simulink model "model"  (R2023b)
settings: Solver=VariableStepAuto  StartTime=0.0  StopTime=10.0  RelTol=1e-3
undefined symbols (not defined in the file): DiscIntNeverNeededParam, Newton, Raphson
libraries: simulink x77, slpidlib x18
(part 3 of 3)

== system model/cfblk32/cfblk14 ==
  cfblk1 : Inport
  cfblk9 : Inport  Port=2
  cfblk10 : Inport  Port=3
  cfblk11 : Inport  Port=4
  cfblk15 : Delay  SampleTime=1
  cfblk3 : simulink/Discrete/Transfer Fcn Lead or Lag  PoleZ=0.95  ZeroZ=0.75  ICPrevOutput=0.0  ICPrevInput=0.0  DoSatur=off
  cfblk4 : slpidlib/PID Controller (2DOF)  Controller=PID  Form=Parallel  TimeDomain=Discrete-time  UseExternalTs=off  SampleTime=1  IntegratorMethod=Forward Euler  FilterMethod=Forward Euler  ControllerParametersSource=internal  P=1  I=1  UseKiTs=off  D=0  N=100  UseFilter=on  b=1  c=1  TunerSelectOption=Transfer Function Based (PID Tuner App)  InitialConditionSource=internal  InitialConditionForIntegrator=0  InitialConditionForFilter=0  DifferentiatorICPrevScaledInput=0  ExternalReset=none  TrackingMode=off  Kt=1  LimitOutput=off  SatLimitsSource=internal  UpperSaturationLimit=inf  LowerSaturationLimit=-inf  LinearizeAsGain=off  AntiWindupMode=none  Kb=1  LimitIntegrator=off  UpperIntegratorSaturationLimit=inf  LowerIntegratorSaturationLimit=-inf  POutMin=[]  POutMax=[]  IOutMin=[]  IOutMax=[]  DOutMin=[]  DOutMax=[]  NOutMin=[]  NOutMax=[]  bOutMin=[]  bOutMax=[]  cOutMin=[]  cOutMax=[]  SumOutMin=[]  SumOutMax=[]  SaturationOutMin=[]  SaturationOutMax=[]  PParamMin=[]  PParamMax=[]  IParamMin=[]  IParamMax=[]  DParamMin=[]  DParamMax=[]  NParamMin=[]  NParamMax=[]  bParamMin=[]  bParamMax=[]  cParamMin=[]  cParamMax=[]  KbParamMin=[]  KbParamMax=[]  KtParamMin=[]  KtParamMax=[]  KbOutMin=[]  KbOutMax=[]  KtOutMin=[]  KtOutMax=[]  IntegratorOutMin=[]  IntegratorOutMax=[]  FilterOutMin=[]  FilterOutMax=[]  SumI1OutMin=[]  SumI1OutMax=[]  SumI2OutMin=[]  SumI2OutMax=[]  SumI3OutMin=[]  SumI3OutMax=[]  SumI4OutMin=[]  SumI4OutMax=[]  SumDOutMin=[]  SumDOutMax=[]  Sum1OutMin=[]  Sum1OutMax=[]  Sum2OutMin=[]  Sum2OutMax=[]  Sum3OutMin=[]  Sum3OutMax=[]  DifferentiatorOutMin=[]  DifferentiatorOutMax=[]  FilterDiffOutCoefMin=[]  FilterDiffOutCoefMax=[]  ReciprocalOutMin=[]  ReciprocalOutMax=[]  SumDenOutMin=[]  SumDenOutMax=[]  SumNumOutMin=[]  SumNumOutMax=[]  DivideOutMin=[]  DivideOutMax=[]  UdiffTsProdOutMin=[]  UdiffTsProdOutMax=[]  NTsProdOutMin=[]  NTsProdOutMax=[]  UintegralTsProdOutMin=[]  UintegralTsProdOutMax=[]  UngainTsProdOutMin=[]  UngainTsProdOutMax=[]  ClampingZeroOutDataTypeStr=Inherit: Inherit via back propagation  ClampingZeroOutMin=[]  ClampingZeroOutMax=[]  FilterDenConstantOutDataTypeStr=Inherit: Inherit via back propagation  FilterDenConstantOutMin=[]  FilterDenConstantOutMax=[]  PCopyOutDataTypeStr=Inherit: Inherit via back propagation  PCopyOutMin=[]  PCopyOutMax=[]  NCopyOutDataTypeStr=Inherit: Inherit via back propagation  NCopyOutMin=[]  NCopyOutMax=[]  IntegratorContinuousStateAttributes=''  IntegratorStateMustResolveToSignalObject=off  IntegratorRTWStateStorageClass=Auto  FilterContinuousStateAttributes=''  FilterStateMustResolveToSignalObject=off  FilterRTWStateStorageClass=Auto  ParallelPVariant=InternalParameters  IdealPVariant=Disabled  IVariant=InternalParameters  DVariant=InternalParameters  bVariant=InternalParameters  cVariant=InternalParameters  IntegratorVariant=Discrete  SatVariant=Disabled  AWVariant=Passthrough  PCopyVariant=Disabled  TRVariant=Disabled  FdbkBlocksVariant=Forward  IdealPFdbkVariant=Disabled  SatFdbkVariant=Disabled  DerivativeFilterVariant=ForwardEulerFilter  NVariant=InternalParameters  NCopyVariant=Disabled  FilterICVariant=InternalICsFilter  IntegratorICVariant=InternalICs  ExternalResetVariant=Disabled  TRSumVariant=Passthrough  SumFdbkVariant=Disabled  SumVariant=Sum_PID  TsampFilterVariant=InternalTs  TsampNgainVariant=Passthrough  TsampIntegralVariant=Disabled_SignalSpec  ExternalSaturationOutDataTypeStr=Inherit: Same as second input
      settings: LibrarySourceBlock=simulink/Discrete/Discrete PID Controller (2DOF)
  cfblk5 : Sin  TimeSource=Use external signal  SampleTime=0
  cfblk6 : Math  Operator=transpose
  cfblk7 : Product
  cfblk8 : Constant  Value=[-199593818.818905]  SampleTime=1
  cfblk2 : Outport
  cfblk12 : Outport  Port=2
  cfblk13 : Outport  Port=3
  cfblk14 : Outport  Port=4
  wires:
  cfblk8/1 -> cfblk2/1
  cfblk6/1 -> cfblk5/1, cfblk7/2
  cfblk5/1 -> cfblk14/1
  cfblk1/1 -> cfblk13/1
  cfblk11/1 -> cfblk12/1
  cfblk9/1 -> cfblk4/1
  cfblk4/1 -> cfblk7/1
  cfblk3/1 -> cfblk6/1
  cfblk10/1 -> cfblk4/2
  cfblk7/1 -> cfblk15/1
  cfblk15/1 -> cfblk3/1

== system model/cfblk32/cfblk8 ==
  cfblk1 : Inport
  cfblk10 : Inport  Port=2
  cfblk11 : Inport  Port=3
  cfblk12 : Inport  Port=4
  cfblk13 : Inport  Port=5
  cfblk14 : Inport  Port=6
  cfblk15 : Delay  SampleTime=1
  cfblk3 : PropagationDelay  SampleTime=1
  cfblk4 : simulink/Discrete/Transfer Fcn Lead or Lag  PoleZ=0.95  ZeroZ=0.75  ICPrevOutput=0.0  ICPrevInput=0.0  DoSatur=off
  cfblk5 : simulink/Discrete/Transfer Fcn First Order  PoleZ=0.95  ICPrevOutput=0.0  DoSatur=off
  cfblk6 : simulink/Discrete/Transfer Fcn Lead or Lag  PoleZ=0.95  ZeroZ=0.75  ICPrevOutput=0.0  ICPrevInput=0.0  DoSatur=off
  cfblk7 : Sum  Inputs=|++
  cfblk8 : Rounding
  cfblk9 : ComplexToRealImag
  cfblk2 : Outport
  wires:
  cfblk12/1 -> cfblk2/1
  cfblk4/1 -> cfblk6/1
  cfblk14/1 -> cfblk8/1
  cfblk11/1 -> cfblk5/1
  cfblk7/1 -> cfblk9/1
  cfblk10/1 -> cfblk4/1
  cfblk5/1 -> cfblk7/1
  cfblk8/1 -> cfblk3/1
  cfblk9/2 -> cfblk3/2
  cfblk9/1 -> cfblk15/1
  cfblk15/1 -> cfblk7/2

== system model/cfblk32/cfblk9 ==
  cfblk1 : Inport
  cfblk5 : Inport  Port=2
  cfblk6 : Inport  Port=3
  cfblk3 : DotProduct  OutDataTypeStr=Inherit: Inherit via internal rule
  cfblk4 : Product  Inputs=**
  cfblk8 : Delay  SampleTime=1
  cfblk2 : Outport
  cfblk7 : Outport  Port=2
  wires:
  cfblk5/1 -> cfblk4/1
  cfblk3/1 -> cfblk4/2, cfblk7/1
  cfblk1/1 -> cfblk2/1
  cfblk6/1 -> cfblk3/1
  cfblk4/1 -> cfblk8/1
  cfblk8/1 -> cfblk3/2

== system model/cfblk35/cfblk10 ==
  cfblk1 : Inport
  cfblk10 : Inport  Port=2
  cfblk11 : Inport  Port=3
  cfblk12 : Inport  Port=4
  cfblk13 : Inport  Port=5
  cfblk3 : DiscreteZeroPole  Poles=[0 0.5]  Gain=1  SampleTime=-1
  cfblk4 : DiscreteStateSpace  SampleTime=-1
  cfblk5 : simulink/Math Operations/Slider Gain  gain=1  low=0  high=2
  cfblk6 : Sin  TimeSource=Use external signal  SampleTime=0
  cfblk7 : Constant  Value=[-112437375.894826]  SampleTime=1
  cfblk8 : Constant  Value=[-453137305.741607]  SampleTime=1
  cfblk9 : Constant  Value=[-741340996.395799]  SampleTime=1
  cfblk2 : Outport
  wires:
  cfblk13/1 -> cfblk6/1
  cfblk5/1 -> cfblk2/1
  cfblk12/1 -> cfblk4/1
  cfblk4/1 -> cfblk3/1
  cfblk6/1 -> cfblk5/1

== system model/cfblk35/cfblk11 ==
  cfblk1 : Inport
  cfblk12 : Inport  Port=2
  cfblk10 : UnaryMinus
  cfblk11 : Squeeze
  cfblk14 : Delay
  cfblk3 : simulink/Discrete/Transfer Fcn Real Zero  ZeroZ=0.75  ICPrevInput=0.0  DoSatur=off
  cfblk4 : DiscreteFir
  cfblk5 : Delay  DelayLengthSource=Input port
      settings: InputPortMap=u0,p1
  cfblk6 : DiscreteStateSpace  SampleTime=-1
  cfblk7 : simulink/Discrete/Transfer Fcn First Order  PoleZ=0.95  ICPrevOutput=0.0  DoSatur=off
  cfblk8 : Reshape
  cfblk9 : simulink/Math Operations/Slider Gain  gain=1  low=0  high=2
  cfblk2 : Outport
  cfblk13 : Outport  Port=2
  wires:
  cfblk4/1 -> cfblk8/1
  cfblk8/1 -> cfblk2/1
  cfblk1/1 -> cfblk10/1
  cfblk3/1 -> cfblk5/1
  cfblk10/1 -> cfblk4/1
  cfblk7/1 -> cfblk9/1
  cfblk11/1 -> cfblk13/1, cfblk6/1
  cfblk12/1 -> cfblk7/1
  cfblk9/1 -> cfblk11/1
  cfblk6/1 -> cfblk5/2
  cfblk5/1 -> cfblk14/1
  cfblk14/1 -> cfblk3/1

== system model/cfblk35/cfblk14 ==
  cfblk1 : Inport
  cfblk5 : Inport  Port=2
  cfblk6 : Inport  Port=3
  Action Port : ActionPort  ActionPortLabel=if(u1 >= 0)
  cfblk3 : DiscreteZeroPole  Poles=[0 0.5]  Gain=1  SampleTime=-1
  cfblk4 : Signum
  cfblk2 : Outport
  cfblk7 : Outport  Port=2
  wires:
  cfblk4/1 -> cfblk3/1
  cfblk5/1 -> cfblk7/1
  cfblk1/1 -> cfblk2/1
  cfblk6/1 -> cfblk4/1

== system model/cfblk35/cfblk15 ==
  cfblk1 : Inport
  Action Port : ActionPort  ActionPortLabel=else
  cfblk10 : Signum
  cfblk11 : Math
  cfblk12 : Bias  Bias=[228101489.768927]  SaturateOnIntegerOverflow=off
  cfblk13 : Constant  Value=[208020800.146715]  SampleTime=1
  cfblk16 : Delay
  cfblk3 : DiscreteStateSpace  SampleTime=-1
  cfblk4 : slpidlib/PID Controller (2DOF)  Controller=PID  Form=Parallel  TimeDomain=Discrete-time  UseExternalTs=off  SampleTime=-1  IntegratorMethod=Forward Euler  FilterMethod=Forward Euler  ControllerParametersSource=internal  P=1  I=1  UseKiTs=off  D=0  N=100  UseFilter=on  b=1  c=1  TunerSelectOption=Transfer Function Based (PID Tuner App)  InitialConditionSource=internal  InitialConditionForIntegrator=0  InitialConditionForFilter=0  DifferentiatorICPrevScaledInput=0  ExternalReset=none  TrackingMode=off  Kt=1  LimitOutput=off  SatLimitsSource=internal  UpperSaturationLimit=inf  LowerSaturationLimit=-inf  LinearizeAsGain=off  AntiWindupMode=none  Kb=1  LimitIntegrator=off  UpperIntegratorSaturationLimit=inf  LowerIntegratorSaturationLimit=-inf  POutMin=[]  POutMax=[]  IOutMin=[]  IOutMax=[]  DOutMin=[]  DOutMax=[]  NOutMin=[]  NOutMax=[]  bOutMin=[]  bOutMax=[]  cOutMin=[]  cOutMax=[]  SumOutMin=[]  SumOutMax=[]  SaturationOutMin=[]  SaturationOutMax=[]  PParamMin=[]  PParamMax=[]  IParamMin=[]  IParamMax=[]  DParamMin=[]  DParamMax=[]  NParamMin=[]  NParamMax=[]  bParamMin=[]  bParamMax=[]  cParamMin=[]  cParamMax=[]  KbParamMin=[]  KbParamMax=[]  KtParamMin=[]  KtParamMax=[]  KbOutMin=[]  KbOutMax=[]  KtOutMin=[]  KtOutMax=[]  IntegratorOutMin=[]  IntegratorOutMax=[]  FilterOutMin=[]  FilterOutMax=[]  SumI1OutMin=[]  SumI1OutMax=[]  SumI2OutMin=[]  SumI2OutMax=[]  SumI3OutMin=[]  SumI3OutMax=[]  SumI4OutMin=[]  SumI4OutMax=[]  SumDOutMin=[]  SumDOutMax=[]  Sum1OutMin=[]  Sum1OutMax=[]  Sum2OutMin=[]  Sum2OutMax=[]  Sum3OutMin=[]  Sum3OutMax=[]  DifferentiatorOutMin=[]  DifferentiatorOutMax=[]  FilterDiffOutCoefMin=[]  FilterDiffOutCoefMax=[]  ReciprocalOutMin=[]  ReciprocalOutMax=[]  SumDenOutMin=[]  SumDenOutMax=[]  SumNumOutMin=[]  SumNumOutMax=[]  DivideOutMin=[]  DivideOutMax=[]  UdiffTsProdOutMin=[]  UdiffTsProdOutMax=[]  NTsProdOutMin=[]  NTsProdOutMax=[]  UintegralTsProdOutMin=[]  UintegralTsProdOutMax=[]  UngainTsProdOutMin=[]  UngainTsProdOutMax=[]  ClampingZeroOutDataTypeStr=Inherit: Inherit via back propagation  ClampingZeroOutMin=[]  ClampingZeroOutMax=[]  FilterDenConstantOutDataTypeStr=Inherit: Inherit via back propagation  FilterDenConstantOutMin=[]  FilterDenConstantOutMax=[]  PCopyOutDataTypeStr=Inherit: Inherit via back propagation  PCopyOutMin=[]  PCopyOutMax=[]  NCopyOutDataTypeStr=Inherit: Inherit via back propagation  NCopyOutMin=[]  NCopyOutMax=[]  IntegratorContinuousStateAttributes=''  IntegratorStateMustResolveToSignalObject=off  IntegratorRTWStateStorageClass=Auto  FilterContinuousStateAttributes=''  FilterStateMustResolveToSignalObject=off  FilterRTWStateStorageClass=Auto  ParallelPVariant=InternalParameters  IdealPVariant=Disabled  IVariant=InternalParameters  DVariant=InternalParameters  bVariant=InternalParameters  cVariant=InternalParameters  IntegratorVariant=Discrete  SatVariant=Disabled  AWVariant=Passthrough  PCopyVariant=Disabled  TRVariant=Disabled  FdbkBlocksVariant=Forward  IdealPFdbkVariant=Disabled  SatFdbkVariant=Disabled  DerivativeFilterVariant=ForwardEulerFilter  NVariant=InternalParameters  NCopyVariant=Disabled  FilterICVariant=InternalICsFilter  IntegratorICVariant=InternalICs  ExternalResetVariant=Disabled  TRSumVariant=Passthrough  SumFdbkVariant=Disabled  SumVariant=Sum_PID  TsampFilterVariant=InternalTs  TsampNgainVariant=Passthrough  TsampIntegralVariant=Disabled_SignalSpec  ExternalSaturationOutDataTypeStr=Inherit: Same as second input
      settings: LibrarySourceBlock=simulink/Discrete/Discrete PID Controller (2DOF)
  cfblk5 : slpidlib/PID Controller  Controller=PID  Form=Parallel  TimeDomain=Discrete-time  UseExternalTs=off  SampleTime=-1  IntegratorMethod=Forward Euler  FilterMethod=Forward Euler  ControllerParametersSource=internal  P=1  I=1  UseKiTs=off  D=0  N=100  UseFilter=on  TunerSelectOption=Transfer Function Based (PID Tuner App)  InitialConditionSource=internal  InitialConditionForIntegrator=0  InitialConditionForFilter=0  DifferentiatorICPrevScaledInput=0  ExternalReset=none  TrackingMode=off  Kt=1  LimitOutput=off  SatLimitsSource=internal  UpperSaturationLimit=inf  LowerSaturationLimit=-inf  LinearizeAsGain=off  AntiWindupMode=none  Kb=1  LimitIntegrator=off  UpperIntegratorSaturationLimit=inf  LowerIntegratorSaturationLimit=-inf  POutMin=[]  POutMax=[]  IOutMin=[]  IOutMax=[]  DOutMin=[]  DOutMax=[]  NOutMin=[]  NOutMax=[]  SumOutMin=[]  SumOutMax=[]  SaturationOutMin=[]  SaturationOutMax=[]  PParamMin=[]  PParamMax=[]  IParamMin=[]  IParamMax=[]  DParamMin=[]  DParamMax=[]  NParamMin=[]  NParamMax=[]  KbParamMin=[]  KbParamMax=[]  KtParamMin=[]  KtParamMax=[]  KbOutMin=[]  KbOutMax=[]  KtOutMin=[]  KtOutMax=[]  IntegratorOutMin=[]  IntegratorOutMax=[]  FilterOutMin=[]  FilterOutMax=[]  SumI1OutMin=[]  SumI1OutMax=[]  SumI2OutMin=[]  SumI2OutMax=[]  SumI3OutMin=[]  SumI3OutMax=[]  SumI4OutMin=[]  SumI4OutMax=[]  SumDOutMin=[]  SumDOutMax=[]  DifferentiatorOutMin=[]  DifferentiatorOutMax=[]  FilterDiffOutCoefMin=[]  FilterDiffOutCoefMax=[]  ReciprocalOutMin=[]  ReciprocalOutMax=[]  SumDenOutMin=[]  SumDenOutMax=[]  SumNumOutMin=[]  SumNumOutMax=[]  DivideOutMin=[]  DivideOutMax=[]  UdiffTsProdOutMin=[]  UdiffTsProdOutMax=[]  NTsProdOutMin=[]  NTsProdOutMax=[]  UintegralTsProdOutMin=[]  UintegralTsProdOutMax=[]  UngainTsProdOutMin=[]  UngainTsProdOutMax=[]  ClampingZeroOutDataTypeStr=Inherit: Inherit via back propagation  ClampingZeroOutMin=[]  ClampingZeroOutMax=[]  FilterDenConstantOutDataTypeStr=Inherit: Inherit via back propagation  FilterDenConstantOutMin=[]  FilterDenConstantOutMax=[]  PCopyOutDataTypeStr=Inherit: Inherit via back propagation  PCopyOutMin=[]  PCopyOutMax=[]  NCopyOutDataTypeStr=Inherit: Inherit via back propagation  NCopyOutMin=[]  NCopyOutMax=[]  IntegratorContinuousStateAttributes=''  IntegratorStateMustResolveToSignalObject=off  IntegratorRTWStateStorageClass=Auto  FilterContinuousStateAttributes=''  FilterStateMustResolveToSignalObject=off  FilterRTWStateStorageClass=Auto  ParallelPVariant=InternalParameters  IdealPVariant=Disabled  IVariant=InternalParameters  DVariant=InternalParameters  IntegratorVariant=Discrete  SatVariant=Disabled  AWVariant=Passthrough  PCopyVariant=Disabled  TRVariant=Disabled  FdbkBlocksVariant=Forward  IdealPFdbkVariant=Disabled  SatFdbkVariant=Disabled  DerivativeFilterVariant=ForwardEulerFilter  NVariant=InternalParameters  NCopyVariant=Disabled  FilterICVariant=InternalICsFilter  IntegratorICVariant=InternalICs  ExternalResetVariant=Disabled  TRSumVariant=Passthrough  SumFdbkVariant=Disabled  SumVariant=Sum_PID  TsampFilterVariant=InternalTs  TsampNgainVariant=Passthrough  TsampIntegralVariant=Disabled_SignalSpec  ExternalSaturationOutDataTypeStr=Inherit: Same as second input
      settings: LibrarySourceBlock=simulink/Discrete/Discrete PID Controller
  cfblk6 : DiscreteZeroPole  Poles=[0 0.5]  Gain=1  SampleTime=-1
  cfblk7 : UnitDelay  SampleTime=-1  HasFrameUpgradeWarning=on
  cfblk8 : slpidlib/PID Controller  Controller=PID  Form=Parallel  TimeDomain=Discrete-time  UseExternalTs=off  SampleTime=-1  IntegratorMethod=Forward Euler  FilterMethod=Forward Euler  ControllerParametersSource=internal  P=1  I=1  UseKiTs=off  D=0  N=100  UseFilter=on  TunerSelectOption=Transfer Function Based (PID Tuner App)  InitialConditionSource=internal  InitialConditionForIntegrator=0  InitialConditionForFilter=0  DifferentiatorICPrevScaledInput=0  ExternalReset=none  TrackingMode=off  Kt=1  LimitOutput=off  SatLimitsSource=internal  UpperSaturationLimit=inf  LowerSaturationLimit=-inf  LinearizeAsGain=off  AntiWindupMode=none  Kb=1  LimitIntegrator=off  UpperIntegratorSaturationLimit=inf  LowerIntegratorSaturationLimit=-inf  POutMin=[]  POutMax=[]  IOutMin=[]  IOutMax=[]  DOutMin=[]  DOutMax=[]  NOutMin=[]  NOutMax=[]  SumOutMin=[]  SumOutMax=[]  SaturationOutMin=[]  SaturationOutMax=[]  PParamMin=[]  PParamMax=[]  IParamMin=[]  IParamMax=[]  DParamMin=[]  DParamMax=[]  NParamMin=[]  NParamMax=[]  KbParamMin=[]  KbParamMax=[]  KtParamMin=[]  KtParamMax=[]  KbOutMin=[]  KbOutMax=[]  KtOutMin=[]  KtOutMax=[]  IntegratorOutMin=[]  IntegratorOutMax=[]  FilterOutMin=[]  FilterOutMax=[]  SumI1OutMin=[]  SumI1OutMax=[]  SumI2OutMin=[]  SumI2OutMax=[]  SumI3OutMin=[]  SumI3OutMax=[]  SumI4OutMin=[]  SumI4OutMax=[]  SumDOutMin=[]  SumDOutMax=[]  DifferentiatorOutMin=[]  DifferentiatorOutMax=[]  FilterDiffOutCoefMin=[]  FilterDiffOutCoefMax=[]  ReciprocalOutMin=[]  ReciprocalOutMax=[]  SumDenOutMin=[]  SumDenOutMax=[]  SumNumOutMin=[]  SumNumOutMax=[]  DivideOutMin=[]  DivideOutMax=[]  UdiffTsProdOutMin=[]  UdiffTsProdOutMax=[]  NTsProdOutMin=[]  NTsProdOutMax=[]  UintegralTsProdOutMin=[]  UintegralTsProdOutMax=[]  UngainTsProdOutMin=[]  UngainTsProdOutMax=[]  ClampingZeroOutDataTypeStr=Inherit: Inherit via back propagation  ClampingZeroOutMin=[]  ClampingZeroOutMax=[]  FilterDenConstantOutDataTypeStr=Inherit: Inherit via back propagation  FilterDenConstantOutMin=[]  FilterDenConstantOutMax=[]  PCopyOutDataTypeStr=Inherit: Inherit via back propagation  PCopyOutMin=[]  PCopyOutMax=[]  NCopyOutDataTypeStr=Inherit: Inherit via back propagation  NCopyOutMin=[]  NCopyOutMax=[]  IntegratorContinuousStateAttributes=''  IntegratorStateMustResolveToSignalObject=off  IntegratorRTWStateStorageClass=Auto  FilterContinuousStateAttributes=''  FilterStateMustResolveToSignalObject=off  FilterRTWStateStorageClass=Auto  ParallelPVariant=InternalParameters  IdealPVariant=Disabled  IVariant=InternalParameters  DVariant=InternalParameters  IntegratorVariant=Discrete  SatVariant=Disabled  AWVariant=Passthrough  PCopyVariant=Disabled  TRVariant=Disabled  FdbkBlocksVariant=Forward  IdealPFdbkVariant=Disabled  SatFdbkVariant=Disabled  DerivativeFilterVariant=ForwardEulerFilter  NVariant=InternalParameters  NCopyVariant=Disabled  FilterICVariant=InternalICsFilter  IntegratorICVariant=InternalICs  ExternalResetVariant=Disabled  TRSumVariant=Passthrough  SumFdbkVariant=Disabled  SumVariant=Sum_PID  TsampFilterVariant=InternalTs  TsampNgainVariant=Passthrough  TsampIntegralVariant=Disabled_SignalSpec  ExternalSaturationOutDataTypeStr=Inherit: Same as second input
      settings: LibrarySourceBlock=simulink/Discrete/Discrete PID Controller
  cfblk9 : Sqrt  Operator=rSqrt  AlgorithmType=Newton-Raphson
  cfblk2 : Outport
  cfblk14 : Outport  Port=2
  cfblk15 : Outport  Port=3
  wires:
  cfblk6/1 -> cfblk4/1
  cfblk4/1 -> cfblk10/1
  cfblk1/1 -> cfblk5/1, cfblk9/1
  cfblk5/1 -> cfblk15/1, cfblk14/1
  cfblk9/1 -> cfblk2/1
  cfblk13/1 -> cfblk4/2
  cfblk12/1 -> cfblk7/1
  cfblk10/1 -> cfblk11/1
  cfblk8/1 -> cfblk6/1
  cfblk3/1 -> cfblk8/1
  cfblk11/1 -> cfblk12/1
  cfblk7/1 -> cfblk16/1
  cfblk16/1 -> cfblk3/1

== system model/cfblk35/cfblk9 ==
  cfblk1 : Inport
  cfblk8 : Inport  Port=2
  cfblk9 : Inport  Port=3
  cfblk10 : Inport  Port=4
  cfblk3 : PermuteDimensions
  cfblk4 : Sum  Inputs=+-
  cfblk5 : Sin  TimeSource=Use external signal  SampleTime=0
  cfblk6 : Constant  Value=[547262071.975775]  SampleTime=1
  cfblk7 : Constant  Value=[-884998425.678320]  SampleTime=1
  cfblk2 : Outport
  cfblk11 : Outport  Port=2
  wires:
  cfblk5/1 -> cfblk3/1
  cfblk10/1 -> cfblk4/1
  cfblk9/1 -> cfblk5/1
  cfblk1/1 -> cfblk11/1
  cfblk7/1 -> cfblk2/1
  cfblk8/1 -> cfblk4/2

== system model/cfblk36/cfblk6 ==
  cfblk1 : Inport
  cfblk13 : Inport  Port=2
  cfblk10 : simulink/Math Operations/Slider Gain  gain=1  low=0  high=2
  cfblk11 : Polyval  Coefs=[ +2.081618890e-019, -1.441693666e-014, +4.719686976e-010, -8.536869453e-006, +1.621573104e-001, -8.087801117e+001 ]
  cfblk12 : Constant  Value=[-516293650.996945]  SampleTime=1
  cfblk15 : Delay
  cfblk3 : DiscreteZeroPole  Poles=[0 0.5]  Gain=1  SampleTime=-1
  cfblk4 : simulink/Discrete/Transfer Fcn Lead or Lag  PoleZ=0.95  ZeroZ=0.75  ICPrevOutput=0.0  ICPrevInput=0.0  DoSatur=off
  cfblk5 : DiscreteStateSpace  SampleTime=-1
  cfblk6 : ComplexToRealImag
  cfblk7 : Trigonometry
  cfblk8 : Product  Inputs=**
  cfblk9 : PermuteDimensions
  cfblk2 : Outport
  cfblk14 : Outport  Port=2
  wires:
  cfblk11/1 -> cfblk5/1
  cfblk6/1 -> cfblk9/1
  cfblk10/1 -> cfblk7/1
  cfblk12/1 -> cfblk14/1
  cfblk4/1 -> cfblk10/1
  cfblk6/2 -> cfblk3/1
  cfblk1/1 -> cfblk6/1
  cfblk13/1 -> cfblk11/1
  cfblk3/1 -> cfblk2/1
  cfblk9/1 -> cfblk8/1
  cfblk5/1 -> cfblk8/2
  cfblk7/1 -> cfblk15/1
  cfblk15/1 -> cfblk4/1

== system model/cfblk36/cfblk7 ==
  cfblk1 : Inport
  cfblk13 : Inport  Port=2
  cfblk14 : Inport  Port=3
  cfblk10 : ComplexToRealImag
  cfblk11 : Constant  Value=[929504628.332843]  SampleTime=1
  cfblk12 : Constant  Value=[-286290192.988281]  SampleTime=1
  cfblk3 : simulink/Discrete/Transfer Fcn Lead or Lag  PoleZ=0.95  ZeroZ=0.75  ICPrevOutput=0.0  ICPrevInput=0.0  DoSatur=off
  cfblk4 : Reshape
  cfblk5 : Bias  Bias=[-880605367.001001]  SaturateOnIntegerOverflow=off
  cfblk6 : DotProduct  OutDataTypeStr=Inherit: Inherit via internal rule
  cfblk7 : PermuteDimensions
  cfblk8 : simulink/Math Operations/MinMax Running Resettable  Function=min  vinit=0.0
  cfblk9 : Sqrt  Operator=rSqrt  AlgorithmType=Newton-Raphson
  cfblk2 : Outport
  cfblk15 : Outport  Port=2
  wires:
  cfblk1/1 -> cfblk9/1
  cfblk5/1 -> cfblk3/1
  cfblk8/1 -> cfblk2/1
  cfblk14/1 -> cfblk8/1
  cfblk6/1 -> cfblk8/2
  cfblk9/1 -> cfblk6/1
  cfblk11/1 -> cfblk15/1
  cfblk3/1 -> cfblk10/1
  cfblk12/1 -> cfblk7/1
  cfblk7/1 -> cfblk6/2
  cfblk4/1 -> cfblk5/1
  cfblk13/1 -> cfblk4/1

== system model/cfblk36/cfblk8 ==
  cfblk1 : Inport
  cfblk7 : Inport  Port=2
  cfblk8 : Inport  Port=3
  cfblk3 : simulink/Discrete/Transfer Fcn Real Zero  ZeroZ=0.75  ICPrevInput=0.0  DoSatur=off
  cfblk4 : simulink/Discrete/Transfer Fcn Real Zero  ZeroZ=0.75  ICPrevInput=0.0  DoSatur=off
  cfblk5 : Constant  Value=[893736484.888777]  SampleTime=1
  cfblk6 : Constant  Value=[-931401752.986753]  SampleTime=1
  cfblk2 : Outport
  cfblk9 : Outport  Port=2
  wires:
  cfblk3/1 -> cfblk9/1
  cfblk8/1 -> cfblk4/1
  cfblk7/1 -> cfblk2/1
  cfblk6/1 -> cfblk3/1

== system model/cfblk37/cfblk4 ==
  cfblk1 : Inport
  cfblk12 : Inport  Port=2
  cfblk13 : Inport  Port=3
  cfblk14 : Inport  Port=4
  cfblk10 : Constant  Value=[-744076515.280142]  SampleTime=1
  cfblk11 : Constant  Value=[-214790099.930049]  SampleTime=1
  cfblk17 : Delay
  cfblk3 : Delay
  cfblk4 : Reshape
  cfblk5 : UnaryMinus
  cfblk6 : Bias  Bias=[884710916.406855]  SaturateOnIntegerOverflow=off
  cfblk7 : MinMax  Function=max  Inputs=2
  cfblk8 : simulink/Math Operations/Slider Gain  gain=1  low=0  high=2
  cfblk9 : Sqrt  Operator=rSqrt  AlgorithmType=Newton-Raphson
  cfblk2 : Outport
  cfblk15 : Outport  Port=2
  cfblk16 : Outport  Port=3
  wires:
  cfblk12/1 -> cfblk5/1
  cfblk9/1 -> cfblk16/1
  cfblk3/1 -> cfblk15/1
  cfblk6/1 -> cfblk2/1
  cfblk7/1 -> cfblk6/1
  cfblk4/1 -> cfblk8/1
  cfblk10/1 -> cfblk9/1
  cfblk13/1 -> cfblk7/1
  cfblk11/1 -> cfblk7/2
  cfblk5/1 -> cfblk3/1
  cfblk8/1 -> cfblk17/1
  cfblk17/1 -> cfblk4/1

== system model/cfblk37/cfblk5 ==
  cfblk1 : Inport
  cfblk14 : Inport  Port=2
  cfblk10 : Abs  SaturateOnIntegerOverflow=off
  cfblk11 : Sum  Inputs=+
  cfblk12 : Constant  Value=[-34818510.735228]  SampleTime=1
  cfblk13 : Constant  Value=[-645267266.388667]  SampleTime=1
  cfblk3 : Delay  DelayLengthSource=Input port
      settings: InputPortMap=u0,p1
  cfblk4 : simulink/Math Operations/Slider Gain  gain=1  low=0  high=2
  cfblk5 : Squeeze
  cfblk6 : Reshape
  cfblk7 : Signum
  cfblk8 : Sin  TimeSource=Use external signal  SampleTime=0
  cfblk9 : simulink/Math Operations/MinMax Running Resettable  Function=min  vinit=0.0
  cfblk2 : Outport
  cfblk15 : Outport  Port=2
  cfblk16 : Outport  Port=3
  wires:
  cfblk9/1 -> cfblk3/1
  cfblk13/1 -> cfblk10/1
  cfblk3/1 -> cfblk5/1
  cfblk10/1 -> cfblk3/2
  cfblk5/1 -> cfblk2/1
  cfblk11/1 -> cfblk7/1
  cfblk12/1 -> cfblk6/1
  cfblk1/1 -> cfblk11/1
  cfblk14/1 -> cfblk15/1
  cfblk8/1 -> cfblk16/1
  cfblk7/1 -> cfblk8/1
  cfblk6/1 -> cfblk4/1
  cfblk4/1 -> cfblk9/1, cfblk9/2

== system model/cfblk37/cfblk6 ==
  cfblk1 : Inport
  cfblk8 : Inport  Port=2
  cfblk9 : Inport  Port=3
  cfblk10 : Delay
  cfblk3 : Delay  DelayLengthSource=Input port
      settings: InputPortMap=u0,p1
  cfblk4 : simulink/Discrete/Difference  ICPrevInput=0.0  OutMin=[]  OutMax=[]  OutDataTypeStr=Inherit: Inherit via back propagation  OutDataType=fixdt(1, 16)  OutScaling=2^-10  DoSatur=off
  cfblk5 : DiscreteStateSpace  SampleTime=-1
  cfblk6 : Abs  SaturateOnIntegerOverflow=off
  cfblk7 : Constant  Value=[-149473581.259236]  SampleTime=1
  cfblk2 : Outport
  wires:
  cfblk1/1 -> cfblk3/1
  cfblk7/1 -> cfblk4/1
  cfblk9/1 -> cfblk5/1
  cfblk3/1 -> cfblk6/1
  cfblk5/1 -> cfblk2/1
  cfblk6/1 -> cfblk10/1
  cfblk10/1 -> cfblk3/2

== system model/cfblk37/cfblk7 ==
  cfblk1 : Inport
  cfblk5 : Inport  Port=2
  cfblk6 : Inport  Port=3
  cfblk7 : Inport  Port=4
  cfblk3 : simulink/Discrete/Transfer Fcn Lead or Lag  PoleZ=0.95  ZeroZ=0.75  ICPrevOutput=0.0  ICPrevInput=0.0  DoSatur=off
  cfblk4 : Sum
  cfblk2 : Outport
  wires:
  cfblk5/1 -> cfblk4/1
  cfblk6/1 -> cfblk4/2
  cfblk1/1 -> cfblk3/1
  cfblk7/1 -> cfblk2/1

== system model/cfblk38/cfblk10 ==
  cfblk1 : Inport
  cfblk8 : Inport  Port=2
  cfblk3 : Abs  SaturateOnIntegerOverflow=off
  cfblk4 : Sin  TimeSource=Use external signal  SampleTime=0
  cfblk5 : Product  Inputs=**
  cfblk6 : Constant  Value=[-244203584.019798]  SampleTime=1
  cfblk7 : Constant  Value=[-497272579.083426]  SampleTime=1
  cfblk2 : Outport
  cfblk9 : Outport  Port=2
  wires:
  cfblk7/1 -> cfblk3/1
  cfblk6/1 -> cfblk4/1
  cfblk3/1 -> cfblk5/1
  cfblk8/1 -> cfblk2/1
  cfblk4/1 -> cfblk5/2
  cfblk1/1 -> cfblk9/1

== system model/cfblk38/cfblk11 ==
  cfblk1 : Inport
  cfblk9 : Inport  Port=2
  cfblk10 : Inport  Port=3
  cfblk11 : Inport  Port=4
  cfblk12 : Inport  Port=5
  cfblk13 : Inport  Port=6
  cfblk14 : Delay
  cfblk3 : slpidlib/PID Controller  Controller=PID  Form=Parallel  TimeDomain=Discrete-time  UseExternalTs=off  SampleTime=-1  IntegratorMethod=Forward Euler  FilterMethod=Forward Euler  ControllerParametersSource=internal  P=1  I=1  UseKiTs=off  D=0  N=100  UseFilter=on  TunerSelectOption=Transfer Function Based (PID Tuner App)  InitialConditionSource=internal  InitialConditionForIntegrator=0  InitialConditionForFilter=0  DifferentiatorICPrevScaledInput=0  ExternalReset=none  TrackingMode=off  Kt=1  LimitOutput=off  SatLimitsSource=internal  UpperSaturationLimit=inf  LowerSaturationLimit=-inf  LinearizeAsGain=off  AntiWindupMode=none  Kb=1  LimitIntegrator=off  UpperIntegratorSaturationLimit=inf  LowerIntegratorSaturationLimit=-inf  POutMin=[]  POutMax=[]  IOutMin=[]  IOutMax=[]  DOutMin=[]  DOutMax=[]  NOutMin=[]  NOutMax=[]  SumOutMin=[]  SumOutMax=[]  SaturationOutMin=[]  SaturationOutMax=[]  PParamMin=[]  PParamMax=[]  IParamMin=[]  IParamMax=[]  DParamMin=[]  DParamMax=[]  NParamMin=[]  NParamMax=[]  KbParamMin=[]  KbParamMax=[]  KtParamMin=[]  KtParamMax=[]  KbOutMin=[]  KbOutMax=[]  KtOutMin=[]  KtOutMax=[]  IntegratorOutMin=[]  IntegratorOutMax=[]  FilterOutMin=[]  FilterOutMax=[]  SumI1OutMin=[]  SumI1OutMax=[]  SumI2OutMin=[]  SumI2OutMax=[]  SumI3OutMin=[]  SumI3OutMax=[]  SumI4OutMin=[]  SumI4OutMax=[]  SumDOutMin=[]  SumDOutMax=[]  DifferentiatorOutMin=[]  DifferentiatorOutMax=[]  FilterDiffOutCoefMin=[]  FilterDiffOutCoefMax=[]  ReciprocalOutMin=[]  ReciprocalOutMax=[]  SumDenOutMin=[]  SumDenOutMax=[]  SumNumOutMin=[]  SumNumOutMax=[]  DivideOutMin=[]  DivideOutMax=[]  UdiffTsProdOutMin=[]  UdiffTsProdOutMax=[]  NTsProdOutMin=[]  NTsProdOutMax=[]  UintegralTsProdOutMin=[]  UintegralTsProdOutMax=[]  UngainTsProdOutMin=[]  UngainTsProdOutMax=[]  ClampingZeroOutDataTypeStr=Inherit: Inherit via back propagation  ClampingZeroOutMin=[]  ClampingZeroOutMax=[]  FilterDenConstantOutDataTypeStr=Inherit: Inherit via back propagation  FilterDenConstantOutMin=[]  FilterDenConstantOutMax=[]  PCopyOutDataTypeStr=Inherit: Inherit via back propagation  PCopyOutMin=[]  PCopyOutMax=[]  NCopyOutDataTypeStr=Inherit: Inherit via back propagation  NCopyOutMin=[]  NCopyOutMax=[]  IntegratorContinuousStateAttributes=''  IntegratorStateMustResolveToSignalObject=off  IntegratorRTWStateStorageClass=Auto  FilterContinuousStateAttributes=''  FilterStateMustResolveToSignalObject=off  FilterRTWStateStorageClass=Auto  ParallelPVariant=InternalParameters  IdealPVariant=Disabled  IVariant=InternalParameters  DVariant=InternalParameters  IntegratorVariant=Discrete  SatVariant=Disabled  AWVariant=Passthrough  PCopyVariant=Disabled  TRVariant=Disabled  FdbkBlocksVariant=Forward  IdealPFdbkVariant=Disabled  SatFdbkVariant=Disabled  DerivativeFilterVariant=ForwardEulerFilter  NVariant=InternalParameters  NCopyVariant=Disabled  FilterICVariant=InternalICsFilter  IntegratorICVariant=InternalICs  ExternalResetVariant=Disabled  TRSumVariant=Passthrough  SumFdbkVariant=Disabled  SumVariant=Sum_PID  TsampFilterVariant=InternalTs  TsampNgainVariant=Passthrough  TsampIntegralVariant=Disabled_SignalSpec  ExternalSaturationOutDataTypeStr=Inherit: Same as second input
      settings: LibrarySourceBlock=simulink/Discrete/Discrete PID Controller
  cfblk4 : UnitDelay  SampleTime=-1  HasFrameUpgradeWarning=on
  cfblk5 : Rounding
  cfblk6 : Polyval  Coefs=[ +2.081618890e-019, -1.441693666e-014, +4.719686976e-010, -8.536869453e-006, +1.621573104e-001, -8.087801117e+001 ]
  cfblk7 : Sum  Inputs=--
  cfblk8 : Squeeze
  cfblk2 : Outport
  wires:
  cfblk13/1 -> cfblk4/1
  cfblk5/1 -> cfblk8/1
  cfblk6/1 -> cfblk2/1
  cfblk1/1 -> cfblk7/1
  cfblk9/1 -> cfblk7/2
  cfblk4/1 -> cfblk3/1
  cfblk7/1 -> cfblk6/1
  cfblk8/1 -> cfblk14/1
  cfblk14/1 -> cfblk5/1

== system model/cfblk38/cfblk12 ==
  cfblk1 : Inport
  cfblk10 : Inport  Port=2
  cfblk11 : Inport  Port=3
  cfblk15 : Delay
  cfblk3 : Delay  DelayLengthSource=Input port
      settings: InputPortMap=u0,p1
  cfblk4 : Delay  DelayLengthSource=Input port
      settings: InputPortMap=u0,p1
  cfblk5 : simulink/Discrete/Difference  ICPrevInput=0.0  OutMin=[]  OutMax=[]  OutDataTypeStr=Inherit: Inherit via back propagation  OutDataType=fixdt(1, 16)  OutScaling=2^-10  DoSatur=off
  cfblk6 : Delay
  cfblk7 : Squeeze
  cfblk8 : Trigonometry
  cfblk9 : Constant  Value=[685636712.719749]  SampleTime=1
  cfblk2 : Outport
  cfblk12 : Outport  Port=2
  cfblk13 : Outport  Port=3
  cfblk14 : Outport  Port=4
  wires:
  cfblk3/1 -> cfblk7/1
  cfblk10/1 -> cfblk13/1
  cfblk8/1 -> cfblk6/1
  cfblk11/1 -> cfblk8/1
  cfblk4/1 -> cfblk2/1
  cfblk7/1 -> cfblk14/1, cfblk15/1
  cfblk9/1 -> cfblk3/1
  cfblk6/1 -> cfblk5/1, cfblk12/1
  cfblk1/1 -> cfblk4/1
  cfblk5/1 -> cfblk4/2
  cfblk15/1 -> cfblk3/2

== system model/cfblk38/cfblk13 ==
  cfblk1 : Inport
  cfblk13 : Inport  Port=2
  cfblk14 : Inport  Port=3
  cfblk15 : Inport  Port=4
  cfblk10 : Polyval  Coefs=[ +2.081618890e-019, -1.441693666e-014, +4.719686976e-010, -8.536869453e-006, +1.621573104e-001, -8.087801117e+001 ]
  cfblk11 : ComplexToRealImag
  cfblk12 : Constant  Value=[836032568.367008]  SampleTime=1
  cfblk3 : DiscreteStateSpace  SampleTime=-1
  cfblk4 : DiscreteStateSpace  SampleTime=-1
  cfblk5 : slpidlib/PID Controller  Controller=PID  Form=Parallel  TimeDomain=Discrete-time  UseExternalTs=off  SampleTime=-1  IntegratorMethod=Forward Euler  FilterMethod=Forward Euler  ControllerParametersSource=internal  P=1  I=1  UseKiTs=off  D=0  N=100  UseFilter=on  TunerSelectOption=Transfer Function Based (PID Tuner App)  InitialConditionSource=internal  InitialConditionForIntegrator=0  InitialConditionForFilter=0  DifferentiatorICPrevScaledInput=0  ExternalReset=none  TrackingMode=off  Kt=1  LimitOutput=off  SatLimitsSource=internal  UpperSaturationLimit=inf  LowerSaturationLimit=-inf  LinearizeAsGain=off  AntiWindupMode=none  Kb=1  LimitIntegrator=off  UpperIntegratorSaturationLimit=inf  LowerIntegratorSaturationLimit=-inf  POutMin=[]  POutMax=[]  IOutMin=[]  IOutMax=[]  DOutMin=[]  DOutMax=[]  NOutMin=[]  NOutMax=[]  SumOutMin=[]  SumOutMax=[]  SaturationOutMin=[]  SaturationOutMax=[]  PParamMin=[]  PParamMax=[]  IParamMin=[]  IParamMax=[]  DParamMin=[]  DParamMax=[]  NParamMin=[]  NParamMax=[]  KbParamMin=[]  KbParamMax=[]  KtParamMin=[]  KtParamMax=[]  KbOutMin=[]  KbOutMax=[]  KtOutMin=[]  KtOutMax=[]  IntegratorOutMin=[]  IntegratorOutMax=[]  FilterOutMin=[]  FilterOutMax=[]  SumI1OutMin=[]  SumI1OutMax=[]  SumI2OutMin=[]  SumI2OutMax=[]  SumI3OutMin=[]  SumI3OutMax=[]  SumI4OutMin=[]  SumI4OutMax=[]  SumDOutMin=[]  SumDOutMax=[]  DifferentiatorOutMin=[]  DifferentiatorOutMax=[]  FilterDiffOutCoefMin=[]  FilterDiffOutCoefMax=[]  ReciprocalOutMin=[]  ReciprocalOutMax=[]  SumDenOutMin=[]  SumDenOutMax=[]  SumNumOutMin=[]  SumNumOutMax=[]  DivideOutMin=[]  DivideOutMax=[]  UdiffTsProdOutMin=[]  UdiffTsProdOutMax=[]  NTsProdOutMin=[]  NTsProdOutMax=[]  UintegralTsProdOutMin=[]  UintegralTsProdOutMax=[]  UngainTsProdOutMin=[]  UngainTsProdOutMax=[]  ClampingZeroOutDataTypeStr=Inherit: Inherit via back propagation  ClampingZeroOutMin=[]  ClampingZeroOutMax=[]  FilterDenConstantOutDataTypeStr=Inherit: Inherit via back propagation  FilterDenConstantOutMin=[]  FilterDenConstantOutMax=[]  PCopyOutDataTypeStr=Inherit: Inherit via back propagation  PCopyOutMin=[]  PCopyOutMax=[]  NCopyOutDataTypeStr=Inherit: Inherit via back propagation  NCopyOutMin=[]  NCopyOutMax=[]  IntegratorContinuousStateAttributes=''  IntegratorStateMustResolveToSignalObject=off  IntegratorRTWStateStorageClass=Auto  FilterContinuousStateAttributes=''  FilterStateMustResolveToSignalObject=off  FilterRTWStateStorageClass=Auto  ParallelPVariant=InternalParameters  IdealPVariant=Disabled  IVariant=InternalParameters  DVariant=InternalParameters  IntegratorVariant=Discrete  SatVariant=Disabled  AWVariant=Passthrough  PCopyVariant=Disabled  TRVariant=Disabled  FdbkBlocksVariant=Forward  IdealPFdbkVariant=Disabled  SatFdbkVariant=Disabled  DerivativeFilterVariant=ForwardEulerFilter  NVariant=InternalParameters  NCopyVariant=Disabled  FilterICVariant=InternalICsFilter  IntegratorICVariant=InternalICs  ExternalResetVariant=Disabled  TRSumVariant=Passthrough  SumFdbkVariant=Disabled  SumVariant=Sum_PID  TsampFilterVariant=InternalTs  TsampNgainVariant=Passthrough  TsampIntegralVariant=Disabled_SignalSpec  ExternalSaturationOutDataTypeStr=Inherit: Same as second input
      settings: LibrarySourceBlock=simulink/Discrete/Discrete PID Controller
  cfblk6 : slpidlib/PID Controller (2DOF)  Controller=PID  Form=Parallel  TimeDomain=Discrete-time  UseExternalTs=off  SampleTime=-1  IntegratorMethod=Forward Euler  FilterMethod=Forward Euler  ControllerParametersSource=internal  P=1  I=1  UseKiTs=off  D=0  N=100  UseFilter=on  b=1  c=1  TunerSelectOption=Transfer Function Based (PID Tuner App)  InitialConditionSource=internal  InitialConditionForIntegrator=0  InitialConditionForFilter=0  DifferentiatorICPrevScaledInput=0  ExternalReset=none  TrackingMode=off  Kt=1  LimitOutput=off  SatLimitsSource=internal  UpperSaturationLimit=inf  LowerSaturationLimit=-inf  LinearizeAsGain=off  AntiWindupMode=none  Kb=1  LimitIntegrator=off  UpperIntegratorSaturationLimit=inf  LowerIntegratorSaturationLimit=-inf  POutMin=[]  POutMax=[]  IOutMin=[]  IOutMax=[]  DOutMin=[]  DOutMax=[]  NOutMin=[]  NOutMax=[]  bOutMin=[]  bOutMax=[]  cOutMin=[]  cOutMax=[]  SumOutMin=[]  SumOutMax=[]  SaturationOutMin=[]  SaturationOutMax=[]  PParamMin=[]  PParamMax=[]  IParamMin=[]  IParamMax=[]  DParamMin=[]  DParamMax=[]  NParamMin=[]  NParamMax=[]  bParamMin=[]  bParamMax=[]  cParamMin=[]  cParamMax=[]  KbParamMin=[]  KbParamMax=[]  KtParamMin=[]  KtParamMax=[]  KbOutMin=[]  KbOutMax=[]  KtOutMin=[]  KtOutMax=[]  IntegratorOutMin=[]  IntegratorOutMax=[]  FilterOutMin=[]  FilterOutMax=[]  SumI1OutMin=[]  SumI1OutMax=[]  SumI2OutMin=[]  SumI2OutMax=[]  SumI3OutMin=[]  SumI3OutMax=[]  SumI4OutMin=[]  SumI4OutMax=[]  SumDOutMin=[]  SumDOutMax=[]  Sum1OutMin=[]  Sum1OutMax=[]  Sum2OutMin=[]  Sum2OutMax=[]  Sum3OutMin=[]  Sum3OutMax=[]  DifferentiatorOutMin=[]  DifferentiatorOutMax=[]  FilterDiffOutCoefMin=[]  FilterDiffOutCoefMax=[]  ReciprocalOutMin=[]  ReciprocalOutMax=[]  SumDenOutMin=[]  SumDenOutMax=[]  SumNumOutMin=[]  SumNumOutMax=[]  DivideOutMin=[]  DivideOutMax=[]  UdiffTsProdOutMin=[]  UdiffTsProdOutMax=[]  NTsProdOutMin=[]  NTsProdOutMax=[]  UintegralTsProdOutMin=[]  UintegralTsProdOutMax=[]  UngainTsProdOutMin=[]  UngainTsProdOutMax=[]  ClampingZeroOutDataTypeStr=Inherit: Inherit via back propagation  ClampingZeroOutMin=[]  ClampingZeroOutMax=[]  FilterDenConstantOutDataTypeStr=Inherit: Inherit via back propagation  FilterDenConstantOutMin=[]  FilterDenConstantOutMax=[]  PCopyOutDataTypeStr=Inherit: Inherit via back propagation  PCopyOutMin=[]  PCopyOutMax=[]  NCopyOutDataTypeStr=Inherit: Inherit via back propagation  NCopyOutMin=[]  NCopyOutMax=[]  IntegratorContinuousStateAttributes=''  IntegratorStateMustResolveToSignalObject=off  IntegratorRTWStateStorageClass=Auto  FilterContinuousStateAttributes=''  FilterStateMustResolveToSignalObject=off  FilterRTWStateStorageClass=Auto  ParallelPVariant=InternalParameters  IdealPVariant=Disabled  IVariant=InternalParameters  DVariant=InternalParameters  bVariant=InternalParameters  cVariant=InternalParameters  IntegratorVariant=Discrete  SatVariant=Disabled  AWVariant=Passthrough  PCopyVariant=Disabled  TRVariant=Disabled  FdbkBlocksVariant=Forward  IdealPFdbkVariant=Disabled  SatFdbkVariant=Disabled  DerivativeFilterVariant=ForwardEulerFilter  NVariant=InternalParameters  NCopyVariant=Disabled  FilterICVariant=InternalICsFilter  IntegratorICVariant=InternalICs  ExternalResetVariant=Disabled  TRSumVariant=Passthrough  SumFdbkVariant=Disabled  SumVariant=Sum_PID  TsampFilterVariant=InternalTs  TsampNgainVariant=Passthrough  TsampIntegralVariant=Disabled_SignalSpec  ExternalSaturationOutDataTypeStr=Inherit: Same as second input
      settings: LibrarySourceBlock=simulink/Discrete/Discrete PID Controller (2DOF)
  cfblk7 : Delay
  cfblk8 : DiscreteFir
  cfblk9 : Polyval  Coefs=[ +2.081618890e-019, -1.441693666e-014, +4.719686976e-010, -8.536869453e-006, +1.621573104e-001, -8.087801117e+001 ]
  cfblk2 : Outport
  cfblk16 : Outport  Port=2
  cfblk17 : Outport  Port=3
  wires:
  cfblk9/1 -> cfblk11/1
  cfblk10/1 -> cfblk16/1
  cfblk8/1 -> cfblk10/1
  cfblk4/1 -> cfblk17/1
  cfblk14/1 -> cfblk9/1
  cfblk7/1 -> cfblk5/1
  cfblk1/1 -> cfblk8/1
  cfblk12/1 -> cfblk7/1
  cfblk13/1 -> cfblk2/1
  cfblk15/1 -> cfblk3/1
  cfblk6/1 -> cfblk4/1
  cfblk3/1 -> cfblk6/1
  cfblk11/1 -> cfblk6/2

== system model/cfblk38/cfblk14 ==
  cfblk1 : Inport
  cfblk8 : Inport  Port=2
  cfblk3 : simulink/Discrete/Tapped Delay  vinit=0.0  samptime=-1  NumDelays=1  DelayOrder=Oldest  includeCurrent=off
  cfblk4 : Sqrt  Operator=rSqrt  AlgorithmType=Newton-Raphson
  cfblk5 : DotProduct  OutDataTypeStr=Inherit: Inherit via internal rule
  cfblk6 : Sum  Inputs=+
  cfblk7 : Constant  Value=[-459725490.486942]  SampleTime=1
  cfblk2 : Outport
  wires:
  cfblk7/1 -> cfblk6/1
  cfblk8/1 -> cfblk3/1
  cfblk3/1 -> cfblk5/1
  cfblk4/1 -> cfblk5/2
  cfblk6/1 -> cfblk4/1
  cfblk5/1 -> cfblk2/1

== system model/cfblk38/cfblk15 ==
  cfblk1 : Inport
  cfblk7 : Inport  Port=2
  cfblk3 : simulink/Discrete/Transfer Fcn Lead or Lag  PoleZ=0.95  ZeroZ=0.75  ICPrevOutput=0.0  ICPrevInput=0.0  DoSatur=off
  cfblk4 : Sqrt
  cfblk5 : Sum
  cfblk6 : Product  Inputs=**
  cfblk8 : Delay
  cfblk2 : Outport
  wires:
  cfblk1/1 -> cfblk6/1
  cfblk3/1 -> cfblk5/1
  cfblk7/1 -> cfblk2/1, cfblk5/2
  cfblk6/1 -> cfblk3/1
  cfblk5/1 -> cfblk4/1
  cfblk4/1 -> cfblk8/1
  cfblk8/1 -> cfblk6/2

== system model/cfblk38/cfblk9 ==
  cfblk1 : Inport
  cfblk11 : Inport  Port=2
  cfblk10 : Constant  Value=[914520238.174114]  SampleTime=1
  cfblk13 : Delay
  cfblk3 : simulink/Discrete/Transfer Fcn Real Zero  ZeroZ=0.75  ICPrevInput=0.0  DoSatur=off
  cfblk4 : DiscreteFir
  cfblk5 : Squeeze
  cfblk6 : Bias  Bias=[760130353.807291]  SaturateOnIntegerOverflow=off
  cfblk7 : Product
  cfblk8 : Sum  Inputs=+
  cfblk9 : Polyval  Coefs=[ +2.081618890e-019, -1.441693666e-014, +4.719686976e-010, -8.536869453e-006, +1.621573104e-001, -8.087801117e+001 ]
  cfblk2 : Outport
  cfblk12 : Outport  Port=2
  wires:
  cfblk10/1 -> cfblk8/1
  cfblk4/1 -> cfblk5/1
  cfblk1/1 -> cfblk3/1
  cfblk6/1 -> cfblk7/1
  cfblk9/1 -> cfblk6/1
  cfblk3/1 -> cfblk12/1
  cfblk5/1 -> cfblk9/1
  cfblk8/1 -> cfblk7/2
  cfblk11/1 -> cfblk2/1
  cfblk7/1 -> cfblk13/1
  cfblk13/1 -> cfblk4/1
